simulink model "NCS_Simulation"  (R2019a)
settings: Solver=ode4  StartTime=0.0  StopTime=200  FixedStep=0.004  MaxStep=0.01  RelTol=1e-3
values from neighbouring files (symbols this model uses):
  CAN2EthernetDelay = 0.000    (= 0)    [Parameter.m]
  CycleTime_Sensor = 1/1000    (= 0.001)    [Parameter.m]
  Ethernet2CANDelay = 0.005    [Parameter.m]
  n = 0.001    [Parameter.m]
  nW_ges = 8    [Parameter.m]
  ReferenceDelay = 0.0    (= 0)    [Parameter.m]
undefined symbols (not defined in the file or in its folder): BUSCapacity, controlGate, entity, m, ReadData, ReadSize, v0
libraries: NCS_Library x250, simulink x12
(part 2 of 3)

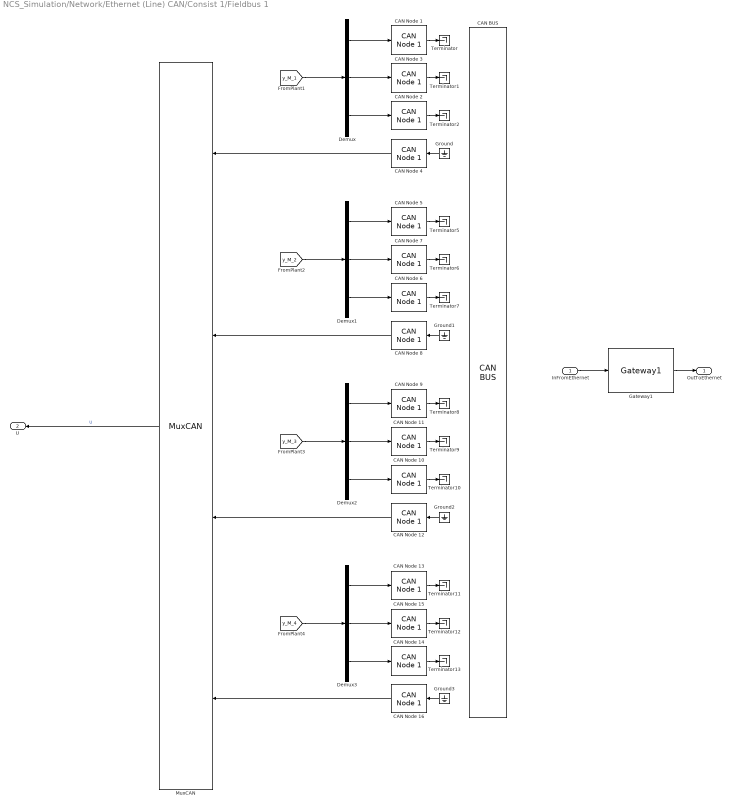
== system NCS_Simulation/Network/Ethernet (Line) CAN/Consist 1/Fieldbus 1 ==
  InFromEthernet : Inport
  CAN BUS : NCS_Library/Network/CAN/CAN BUS  BusID=1  Capacity=500000  LossRate=0.001
  CAN Node 1 : NCS_Library/Network/CAN/CAN Node 1  MsgID=1  IDRange=[1:25]  T_Tx=0.05  SensorType=Position Sensor  MsgSize=8  IDSubscription=[0,0,0,0,0,0,0,0,0,0,0,0,0,0,0,0,0,0,0,0,0,0,0,0,0]  EnableToF=off  ToF=0
  CAN Node 10 : NCS_Library/Network/CAN/CAN Node 1  MsgID=11  IDRange=[1:25]  T_Tx=0.05  SensorType=Acceleration Sensor  MsgSize=8  IDSubscription=[0,0,0,0,0,0,0,0,0,0,0,0,0,0,0,0,0,0,0,0,0,0,0,0,0]  EnableToF=off  ToF=0
  CAN Node 11 : NCS_Library/Network/CAN/CAN Node 1  MsgID=10  IDRange=[1:25]  T_Tx=0.05  SensorType=Velocity Sensor  MsgSize=8  IDSubscription=[0,0,0,0,0,0,0,0,0,0,0,0,0,0,0,0,0,0,0,0,0,0,0,0,0]  EnableToF=off  ToF=0
  CAN Node 12 : NCS_Library/Network/CAN/CAN Node 1  MsgID=12  IDRange=[1:25]  T_Tx=0  SensorType=Actuator  MsgSize=8  IDSubscription=[0,0,0,0,0,0,0,0,0,0,0,0,0,0,0,0,0,0,0,0,0,0,0,0,1]  EnableToF=off  ToF=0
  CAN Node 13 : NCS_Library/Network/CAN/CAN Node 1  MsgID=13  IDRange=[1:25]  T_Tx=0.05  SensorType=Position Sensor  MsgSize=8  IDSubscription=[0,0,0,0,0,0,0,0,0,0,0,0,0,0,0,0,0,0,0,0,0,0,0,0,0]  EnableToF=off  ToF=0
  CAN Node 14 : NCS_Library/Network/CAN/CAN Node 1  MsgID=15  IDRange=[1:25]  T_Tx=0.05  SensorType=Acceleration Sensor  MsgSize=8  IDSubscription=[0,0,0,0,0,0,0,0,0,0,0,0,0,0,0,0,0,0,0,0,0,0,0,0,0]  EnableToF=off  ToF=0
  CAN Node 15 : NCS_Library/Network/CAN/CAN Node 1  MsgID=14  IDRange=[1:25]  T_Tx=0.05  SensorType=Velocity Sensor  MsgSize=8  IDSubscription=[0,0,0,0,0,0,0,0,0,0,0,0,0,0,0,0,0,0,0,0,0,0,0,0,0]  EnableToF=off  ToF=0
  CAN Node 16 : NCS_Library/Network/CAN/CAN Node 1  MsgID=16  IDRange=[1:25]  T_Tx=0  SensorType=Actuator  MsgSize=8  IDSubscription=[0,0,0,0,0,0,0,0,0,0,0,0,0,0,0,0,0,0,0,0,0,0,0,0,1]  EnableToF=off  ToF=0
  CAN Node 2 : NCS_Library/Network/CAN/CAN Node 1  MsgID=3  IDRange=[1:25]  T_Tx=0.05  SensorType=Acceleration Sensor  MsgSize=8  IDSubscription=[0,0,0,0,0,0,0,0,0,0,0,0,0,0,0,0,0,0,0,0,0,0,0,0,0]  EnableToF=off  ToF=0
  CAN Node 3 : NCS_Library/Network/CAN/CAN Node 1  MsgID=2  IDRange=[1:25]  T_Tx=0.05  SensorType=Velocity Sensor  MsgSize=8  IDSubscription=[0,0,0,0,0,0,0,0,0,0,0,0,0,0,0,0,0,0,0,0,0,0,0,0,0]  EnableToF=off  ToF=0
  CAN Node 4 : NCS_Library/Network/CAN/CAN Node 1  MsgID=4  IDRange=[1:25]  T_Tx=0  SensorType=Actuator  MsgSize=8  IDSubscription=[0,0,0,0,0,0,0,0,0,0,0,0,0,0,0,0,0,0,0,0,0,0,0,0,1]  EnableToF=off  ToF=0
  CAN Node 5 : NCS_Library/Network/CAN/CAN Node 1  MsgID=5  IDRange=[1:25]  T_Tx=0.05  SensorType=Position Sensor  MsgSize=8  IDSubscription=[0,0,0,0,0,0,0,0,0,0,0,0,0,0,0,0,0,0,0,0,0,0,0,0,0]  EnableToF=off  ToF=0
  CAN Node 6 : NCS_Library/Network/CAN/CAN Node 1  MsgID=7  IDRange=[1:25]  T_Tx=0.05  SensorType=Acceleration Sensor  MsgSize=8  IDSubscription=[0,0,0,0,0,0,0,0,0,0,0,0,0,0,0,0,0,0,0,0,0,0,0,0,0]  EnableToF=off  ToF=0
  CAN Node 7 : NCS_Library/Network/CAN/CAN Node 1  MsgID=6  IDRange=[1:25]  T_Tx=0.05  SensorType=Velocity Sensor  MsgSize=8  IDSubscription=[0,0,0,0,0,0,0,0,0,0,0,0,0,0,0,0,0,0,0,0,0,0,0,0,0]  EnableToF=off  ToF=0
  CAN Node 8 : NCS_Library/Network/CAN/CAN Node 1  MsgID=8  IDRange=[1:25]  T_Tx=0  SensorType=Actuator  MsgSize=8  IDSubscription=[0,0,0,0,0,0,0,0,0,0,0,0,0,0,0,0,0,0,0,0,0,0,0,0,1]  EnableToF=off  ToF=0
  CAN Node 9 : NCS_Library/Network/CAN/CAN Node 1  MsgID=9  IDRange=[1:25]  T_Tx=0.05  SensorType=Position Sensor  MsgSize=8  IDSubscription=[0,0,0,0,0,0,0,0,0,0,0,0,0,0,0,0,0,0,0,0,0,0,0,0,0]  EnableToF=off  ToF=0
  Demux{,1..3} (4 alike) : Demux  Outputs=3
  Gateway1 : NCS_Library/Network/Gateway/Gateway1  T_Tx=4  MaxNum=8  Address=[111 211]  Destination=[111 200]  Port=1  ReplyAddress=[0 0]  Subscribe=[111 212; 111 213; 0 0; 0 0; 0 0]  Timeout=inf  SDTv2=Disable  SensorType=0  MsgID=25  IDRange=[1:25]  T_Tx_CAN=0.1  MsgSize=8  IDSubscription=[0,1,0,0,0,1,0,0,0,1,0,0,0,1,0,0,0,0,0,0,0,0,0,0,0]  EnableToF=off  ToF=0
  Ground{,1..3} (4 alike) : Ground
  MuxCAN : NCS_Library/Network/Applications/Multiplexer/MuxCAN  SystemSampleTime=-1
  Terminator{,1..2,5..13} (12 alike) : Terminator
  OutToEthernet : Outport
  U : Outport  Port=2
  wires:
  CAN Node 8/1 -> MuxCAN/2
  CAN Node 4/1 -> MuxCAN/1
  Demux/1 -> CAN Node 1/1
  CAN Node 16/1 -> MuxCAN/4
  CAN Node 9/1 -> Terminator8/1
  CAN Node 1/1 -> Terminator/1
  Demux/2 -> CAN Node 3/1
  [y_M_1] -> Demux/1
  Demux3/1 -> CAN Node 13/1
  CAN Node 12/1 -> MuxCAN/3
  Demux2/2 -> CAN Node 11/1
  CAN Node 3/1 -> Terminator1/1
  CAN Node 6/1 -> Terminator7/1
  Ground/1 -> CAN Node 4/1
  CAN Node 5/1 -> Terminator5/1
  Demux/3 -> CAN Node 2/1
  Demux1/3 -> CAN Node 6/1
  Ground3/1 -> CAN Node 16/1
  Ground1/1 -> CAN Node 8/1
  CAN Node 10/1 -> Terminator10/1
  InFromEthernet/1 -> Gateway1/1
  Demux2/1 -> CAN Node 9/1
  CAN Node 11/1 -> Terminator9/1
  CAN Node 13/1 -> Terminator11/1
  Demux2/3 -> CAN Node 10/1
  Demux1/2 -> CAN Node 7/1
  Demux3/2 -> CAN Node 15/1
  CAN Node 14/1 -> Terminator13/1
  Ground2/1 -> CAN Node 12/1
  [y_M_4] -> Demux3/1
  [y_M_3] -> Demux2/1
  Demux1/1 -> CAN Node 5/1
  CAN Node 15/1 -> Terminator12/1
  [y_M_2] -> Demux1/1
  CAN Node 2/1 -> Terminator2/1
  Demux3/3 -> CAN Node 14/1
  CAN Node 7/1 -> Terminator6/1
  MuxCAN/1 -> U/1  "U"
  Gateway1/1 -> OutToEthernet/1

== system NCS_Simulation/Network/Ethernet (Line) CAN/Consist 1/Output Control ==
  <#Receive> : Inport
  Y_M1 : Inport  Port=2
  U : Inport  Port=3
  Y_M2 : Inport  Port=4
  Logical Operator : Logic  Operator=NOT  AllPortsSameDT=off  OutDataTypeStr=boolean
  Mux : NCS_Library/Network/Applications/Multiplexer/Mux  SystemSampleTime=-1
  Switch : Switch  Criteria=u2 > Threshold
  Watch Dog : NCS_Library/Network/Applications/Watch Dog  SystemSampleTime=-1
  Out1 : Outport
  wires:
  Mux/1 -> Out1/1
  Watch Dog/1 -> Logical Operator/1
  U/1 -> Mux/2
  <#Receive>/1 -> Watch Dog/1
  Switch/1 -> Mux/1
  Y_M1/1 -> Switch/1
  Logical Operator/1 -> Switch/2
  Y_M2/1 -> Switch/3

== system NCS_Simulation/Network/Ethernet (Line) CAN/Consist 1/Redundant Device Control ==
  <#Receive> : Inport
  InTx : Inport  Port=2
  Add Constant : Bias  Bias=1
  Display : Display
  Entity Output Switch : EntityOutputSwitch  InputPortMessageModes=m,m  OutputPortMessageModes=m,m  SwitchingCriterion=From control port  SwitchAttributeName=Attribute1
      settings: InputPortMap=u0,u1
  Message Send : MessageSend  OutputPortMessageModes=m
      settings: InputPortMap=u1
  No Failure : EntityTerminator  InputPortMessageModes=m  NumberEntitiesArrived=on
      settings: OutputPortMap=o0
  Watch Dog : NCS_Library/Network/Applications/Watch Dog  SystemSampleTime=-1
  OutTx : Outport
  wires:
  Message Send/1 -> Entity Output Switch/1
  Add Constant/1 -> Message Send/1
  Watch Dog/1 -> Add Constant/1
  No Failure/1 -> Display/1
  <#Receive>/1 -> Watch Dog/1
  Entity Output Switch/1 -> No Failure/1
  InTx/1 -> Entity Output Switch/2
  Entity Output Switch/2 -> OutTx/1

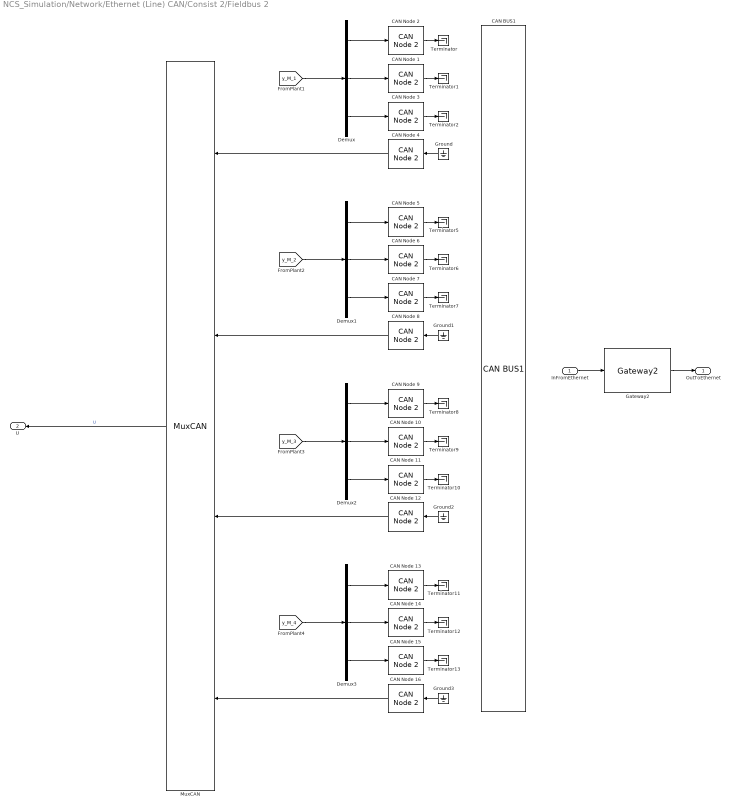
== system NCS_Simulation/Network/Ethernet (Line) CAN/Consist 2/Fieldbus 2 ==
  InFromEthernet : Inport
  CAN BUS1 : NCS_Library/Network/CAN/CAN BUS1  BusID=2  Capacity=500000  LossRate=0.001
  CAN Node 1 : NCS_Library/Network/CAN/CAN Node 2  MsgID=2  IDRange=[1:25]  T_Tx=0.05  SensorType=Velocity Sensor  MsgSize=8  IDSubscription=[0,0,0,0,0,0,0,0,0,0,0,0,0,0,0,0,0,0,0,0,0,0,0,0,0]  EnableToF=off  ToF=0
  CAN Node 10 : NCS_Library/Network/CAN/CAN Node 2  MsgID=10  IDRange=[1:25]  T_Tx=0.05  SensorType=Velocity Sensor  MsgSize=8  IDSubscription=[0,0,0,0,0,0,0,0,0,0,0,0,0,0,0,0,0,0,0,0,0,0,0,0,0]  EnableToF=off  ToF=0
  CAN Node 11 : NCS_Library/Network/CAN/CAN Node 2  MsgID=11  IDRange=[1:25]  T_Tx=0.05  SensorType=Acceleration Sensor  MsgSize=8  IDSubscription=[0,0,0,0,0,0,0,0,0,0,0,0,0,0,0,0,0,0,0,0,0,0,0,0,0]  EnableToF=off  ToF=0
  CAN Node 12 : NCS_Library/Network/CAN/CAN Node 2  MsgID=12  IDRange=[1:25]  T_Tx=0  SensorType=Actuator  MsgSize=8  IDSubscription=[0,0,0,0,0,0,0,0,0,0,0,0,0,0,0,0,0,0,0,0,0,0,0,0,1]  EnableToF=off  ToF=0
  CAN Node 13 : NCS_Library/Network/CAN/CAN Node 2  MsgID=13  IDRange=[1:25]  T_Tx=0.05  SensorType=Position Sensor  MsgSize=8  IDSubscription=[0,0,0,0,0,0,0,0,0,0,0,0,0,0,0,0,0,0,0,0,0,0,0,0,0]  EnableToF=off  ToF=0
  CAN Node 14 : NCS_Library/Network/CAN/CAN Node 2  MsgID=14  IDRange=[1:25]  T_Tx=0.05  SensorType=Velocity Sensor  MsgSize=8  IDSubscription=[0,0,0,0,0,0,0,0,0,0,0,0,0,0,0,0,0,0,0,0,0,0,0,0,0]  EnableToF=off  ToF=0
  CAN Node 15 : NCS_Library/Network/CAN/CAN Node 2  MsgID=15  IDRange=[1:25]  T_Tx=0.05  SensorType=Acceleration Sensor  MsgSize=8  IDSubscription=[0,0,0,0,0,0,0,0,0,0,0,0,0,0,0,0,0,0,0,0,0,0,0,0,0]  EnableToF=off  ToF=0
  CAN Node 16 : NCS_Library/Network/CAN/CAN Node 2  MsgID=16  IDRange=[1:25]  T_Tx=0  SensorType=Actuator  MsgSize=8  IDSubscription=[0,0,0,0,0,0,0,0,0,0,0,0,0,0,0,0,0,0,0,0,0,0,0,0,1]  EnableToF=off  ToF=0
  CAN Node 2 : NCS_Library/Network/CAN/CAN Node 2  MsgID=1  IDRange=[1:25]  T_Tx=0.05  SensorType=Position Sensor  MsgSize=8  IDSubscription=[0,0,0,0,0,0,0,0,0,0,0,0,0,0,0,0,0,0,0,0,0,0,0,0,0]  EnableToF=off  ToF=0
  CAN Node 3 : NCS_Library/Network/CAN/CAN Node 2  MsgID=3  IDRange=[1:25]  T_Tx=0.05  SensorType=Acceleration Sensor  MsgSize=8  IDSubscription=[0,0,0,0,0,0,0,0,0,0,0,0,0,0,0,0,0,0,0,0,0,0,0,0,0]  EnableToF=off  ToF=0
  CAN Node 4 : NCS_Library/Network/CAN/CAN Node 2  MsgID=4  IDRange=[1:25]  T_Tx=0  SensorType=Actuator  MsgSize=8  IDSubscription=[0,0,0,0,0,0,0,0,0,0,0,0,0,0,0,0,0,0,0,0,0,0,0,0,1]  EnableToF=off  ToF=0
  CAN Node 5 : NCS_Library/Network/CAN/CAN Node 2  MsgID=5  IDRange=[1:25]  T_Tx=0.05  SensorType=Position Sensor  MsgSize=8  IDSubscription=[0,0,0,0,0,0,0,0,0,0,0,0,0,0,0,0,0,0,0,0,0,0,0,0,0]  EnableToF=off  ToF=0
  CAN Node 6 : NCS_Library/Network/CAN/CAN Node 2  MsgID=6  IDRange=[1:25]  T_Tx=0.05  SensorType=Velocity Sensor  MsgSize=8  IDSubscription=[0,0,0,0,0,0,0,0,0,0,0,0,0,0,0,0,0,0,0,0,0,0,0,0,0]  EnableToF=off  ToF=0
  CAN Node 7 : NCS_Library/Network/CAN/CAN Node 2  MsgID=7  IDRange=[1:25]  T_Tx=0.05  SensorType=Actuator  MsgSize=8  IDSubscription=[0,0,0,0,0,0,0,0,0,0,0,0,0,0,0,0,0,0,0,0,0,0,0,0,0]  EnableToF=off  ToF=0
  CAN Node 8 : NCS_Library/Network/CAN/CAN Node 2  MsgID=8  IDRange=[1:25]  T_Tx=0  SensorType=Actuator  MsgSize=8  IDSubscription=[0,0,0,0,0,0,0,0,0,0,0,0,0,0,0,0,0,0,0,0,0,0,0,0,1]  EnableToF=off  ToF=0
  CAN Node 9 : NCS_Library/Network/CAN/CAN Node 2  MsgID=9  IDRange=[1:25]  T_Tx=0.05  SensorType=Position Sensor  MsgSize=8  IDSubscription=[0,0,0,0,0,0,0,0,0,0,0,0,0,0,0,0,0,0,0,0,0,0,0,0,0]  EnableToF=off  ToF=0
  Demux{,1..3} (4 alike) : Demux  Outputs=3
  Gateway2 : NCS_Library/Network/Gateway/Gateway2  T_Tx=4  MaxNum=8  Address=[112 211]  Destination=[112 200]  Port=1  ReplyAddress=[0 0]  Subscribe=[112 212; 112 213; 0 0; 0 0; 0 0]  Timeout=inf  SDTv2=Disable  SensorType=0  MsgID=25  IDRange=[1:25]  T_Tx_CAN=0.1  MsgSize=8  IDSubscription=[0,1,0,0,0,1,0,0,0,1,0,0,0,1,0,0,0,0,0,0,0,0,0,0,0]  EnableToF=off  ToF=0
  Ground{,1..3} (4 alike) : Ground
  MuxCAN : NCS_Library/Network/Applications/Multiplexer/MuxCAN  SystemSampleTime=-1
  Terminator{,1..2,5..13} (12 alike) : Terminator
  OutToEthernet : Outport
  U : Outport  Port=2
  wires:
  MuxCAN/1 -> U/1  "U"
  Demux1/2 -> CAN Node 6/1
  Demux/3 -> CAN Node 3/1
  [y_M_2] -> Demux1/1
  Demux3/2 -> CAN Node 14/1
  [y_M_3] -> Demux2/1
  [y_M_4] -> Demux3/1
  Demux3/3 -> CAN Node 15/1
  Demux3/1 -> CAN Node 13/1
  Demux2/2 -> CAN Node 10/1
  InFromEthernet/1 -> Gateway2/1
  Demux2/3 -> CAN Node 11/1
  Demux1/1 -> CAN Node 5/1
  Demux1/3 -> CAN Node 7/1
  Demux/2 -> CAN Node 1/1
  Ground2/1 -> CAN Node 12/1
  [y_M_1] -> Demux/1
  CAN Node 2/1 -> Terminator/1
  Demux2/1 -> CAN Node 9/1
  Ground3/1 -> CAN Node 16/1
  Demux/1 -> CAN Node 2/1
  Ground/1 -> CAN Node 4/1
  Ground1/1 -> CAN Node 8/1
  CAN Node 1/1 -> Terminator1/1
  CAN Node 3/1 -> Terminator2/1
  CAN Node 4/1 -> MuxCAN/1
  CAN Node 5/1 -> Terminator5/1
  CAN Node 6/1 -> Terminator6/1
  CAN Node 7/1 -> Terminator7/1
  CAN Node 8/1 -> MuxCAN/2
  CAN Node 9/1 -> Terminator8/1
  CAN Node 10/1 -> Terminator9/1
  CAN Node 11/1 -> Terminator10/1
  CAN Node 12/1 -> MuxCAN/3
  CAN Node 13/1 -> Terminator11/1
  CAN Node 14/1 -> Terminator12/1
  CAN Node 15/1 -> Terminator13/1
  CAN Node 16/1 -> MuxCAN/4
  Gateway2/1 -> OutToEthernet/1

== system NCS_Simulation/Network/Ethernet (Line) CAN/Consist 2/Output Control ==
  <#Receive> : Inport
  Y_M1 : Inport  Port=2
  U : Inport  Port=3
  Y_M2 : Inport  Port=4
  Logical Operator : Logic  Operator=NOT  AllPortsSameDT=off  OutDataTypeStr=boolean
  MATLAB Function : MATLAB Function  TreatAsAtomicUnit=on
  Switch : Switch  Criteria=u2 > Threshold
  Watch Dog : NCS_Library/Network/Applications/Watch Dog  SystemSampleTime=-1
  Out1 : Outport
  wires:
  Y_M2/1 -> Switch/3
  Logical Operator/1 -> Switch/2
  Y_M1/1 -> Switch/1
  Switch/1 -> MATLAB Function/1(in_Y_M)
  <#Receive>/1 -> Watch Dog/1
  U/1 -> MATLAB Function/2(in_U)
  Watch Dog/1 -> Logical Operator/1
  MATLAB Function/1(out) -> Out1/1

== system NCS_Simulation/Network/Ethernet (Line) CAN/Consist 2/Redundant Device Control ==
  <#Receive> : Inport
  InTx : Inport  Port=2
  Add Constant : Bias  Bias=1
  Display : Display
  Entity Output Switch : EntityOutputSwitch  InputPortMessageModes=m,m  OutputPortMessageModes=m,m  SwitchingCriterion=From control port  SwitchAttributeName=Attribute1
      settings: InputPortMap=u0,u1
  Message Send : MessageSend  OutputPortMessageModes=m
      settings: InputPortMap=u1
  No Failure : EntityTerminator  InputPortMessageModes=m  NumberEntitiesArrived=on
      settings: OutputPortMap=o0
  Watch Dog : NCS_Library/Network/Applications/Watch Dog  SystemSampleTime=-1
  OutTx : Outport
  wires:
  Entity Output Switch/2 -> OutTx/1
  InTx/1 -> Entity Output Switch/2
  Entity Output Switch/1 -> No Failure/1
  <#Receive>/1 -> Watch Dog/1
  No Failure/1 -> Display/1
  Watch Dog/1 -> Add Constant/1
  Add Constant/1 -> Message Send/1
  Message Send/1 -> Entity Output Switch/1

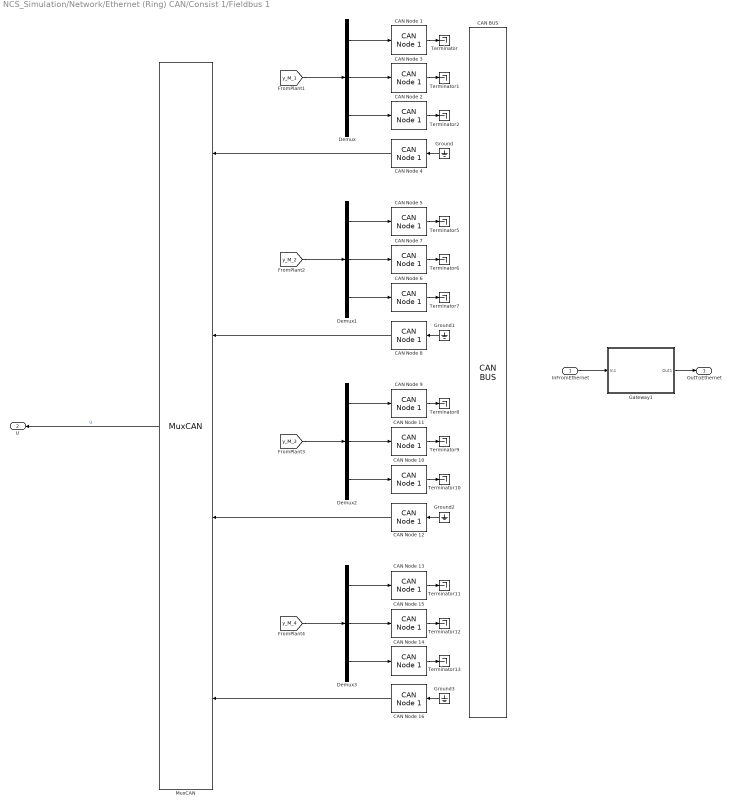
== system NCS_Simulation/Network/Ethernet (Ring) CAN/Consist 1/Fieldbus 1 ==
  InFromEthernet : Inport
  CAN BUS : NCS_Library/Network/CAN/CAN BUS  BusID=1  Capacity=500000  LossRate=0.001
  CAN Node 1 : NCS_Library/Network/CAN/CAN Node 1  MsgID=1  IDRange=[1:25]  T_Tx=0.05  SensorType=Position Sensor  MsgSize=8  IDSubscription=[0,0,0,0,0,0,0,0,0,0,0,0,0,0,0,0,0,0,0,0,0,0,0,0,0]  EnableToF=off  ToF=0
  CAN Node 10 : NCS_Library/Network/CAN/CAN Node 1  MsgID=11  IDRange=[1:25]  T_Tx=0.05  SensorType=Acceleration Sensor  MsgSize=8  IDSubscription=[0,0,0,0,0,0,0,0,0,0,0,0,0,0,0,0,0,0,0,0,0,0,0,0,0]  EnableToF=off  ToF=0
  CAN Node 11 : NCS_Library/Network/CAN/CAN Node 1  MsgID=10  IDRange=[1:25]  T_Tx=0.05  SensorType=Velocity Sensor  MsgSize=8  IDSubscription=[0,0,0,0,0,0,0,0,0,0,0,0,0,0,0,0,0,0,0,0,0,0,0,0,0]  EnableToF=off  ToF=0
  CAN Node 12 : NCS_Library/Network/CAN/CAN Node 1  MsgID=12  IDRange=[1:25]  T_Tx=0  SensorType=Actuator  MsgSize=8  IDSubscription=[0,0,0,0,0,0,0,0,0,0,0,0,0,0,0,0,0,0,0,0,0,0,0,0,1]  EnableToF=off  ToF=0
  CAN Node 13 : NCS_Library/Network/CAN/CAN Node 1  MsgID=13  IDRange=[1:25]  T_Tx=0.05  SensorType=Position Sensor  MsgSize=8  IDSubscription=[0,0,0,0,0,0,0,0,0,0,0,0,0,0,0,0,0,0,0,0,0,0,0,0,0]  EnableToF=off  ToF=0
  CAN Node 14 : NCS_Library/Network/CAN/CAN Node 1  MsgID=15  IDRange=[1:25]  T_Tx=0.05  SensorType=Acceleration Sensor  MsgSize=8  IDSubscription=[0,0,0,0,0,0,0,0,0,0,0,0,0,0,0,0,0,0,0,0,0,0,0,0,0]  EnableToF=off  ToF=0
  CAN Node 15 : NCS_Library/Network/CAN/CAN Node 1  MsgID=14  IDRange=[1:25]  T_Tx=0.05  SensorType=Velocity Sensor  MsgSize=8  IDSubscription=[0,0,0,0,0,0,0,0,0,0,0,0,0,0,0,0,0,0,0,0,0,0,0,0,0]  EnableToF=off  ToF=0
  CAN Node 16 : NCS_Library/Network/CAN/CAN Node 1  MsgID=16  IDRange=[1:25]  T_Tx=0  SensorType=Actuator  MsgSize=8  IDSubscription=[0,0,0,0,0,0,0,0,0,0,0,0,0,0,0,0,0,0,0,0,0,0,0,0,1]  EnableToF=off  ToF=0
  CAN Node 2 : NCS_Library/Network/CAN/CAN Node 1  MsgID=3  IDRange=[1:25]  T_Tx=0.05  SensorType=Acceleration Sensor  MsgSize=8  IDSubscription=[0,0,0,0,0,0,0,0,0,0,0,0,0,0,0,0,0,0,0,0,0,0,0,0,0]  EnableToF=off  ToF=0
  CAN Node 3 : NCS_Library/Network/CAN/CAN Node 1  MsgID=2  IDRange=[1:25]  T_Tx=0.05  SensorType=Velocity Sensor  MsgSize=8  IDSubscription=[0,0,0,0,0,0,0,0,0,0,0,0,0,0,0,0,0,0,0,0,0,0,0,0,0]  EnableToF=off  ToF=0
  CAN Node 4 : NCS_Library/Network/CAN/CAN Node 1  MsgID=4  IDRange=[1:25]  T_Tx=0  SensorType=Actuator  MsgSize=8  IDSubscription=[0,0,0,0,0,0,0,0,0,0,0,0,0,0,0,0,0,0,0,0,0,0,0,0,1]  EnableToF=off  ToF=0
  CAN Node 5 : NCS_Library/Network/CAN/CAN Node 1  MsgID=5  IDRange=[1:25]  T_Tx=0.05  SensorType=Position Sensor  MsgSize=8  IDSubscription=[0,0,0,0,0,0,0,0,0,0,0,0,0,0,0,0,0,0,0,0,0,0,0,0,0]  EnableToF=off  ToF=0
  CAN Node 6 : NCS_Library/Network/CAN/CAN Node 1  MsgID=7  IDRange=[1:25]  T_Tx=0.05  SensorType=Acceleration Sensor  MsgSize=8  IDSubscription=[0,0,0,0,0,0,0,0,0,0,0,0,0,0,0,0,0,0,0,0,0,0,0,0,0]  EnableToF=off  ToF=0
  CAN Node 7 : NCS_Library/Network/CAN/CAN Node 1  MsgID=6  IDRange=[1:25]  T_Tx=0.05  SensorType=Velocity Sensor  MsgSize=8  IDSubscription=[0,0,0,0,0,0,0,0,0,0,0,0,0,0,0,0,0,0,0,0,0,0,0,0,0]  EnableToF=off  ToF=0
  CAN Node 8 : NCS_Library/Network/CAN/CAN Node 1  MsgID=8  IDRange=[1:25]  T_Tx=0  SensorType=Actuator  MsgSize=8  IDSubscription=[0,0,0,0,0,0,0,0,0,0,0,0,0,0,0,0,0,0,0,0,0,0,0,0,1]  EnableToF=off  ToF=0
  CAN Node 9 : NCS_Library/Network/CAN/CAN Node 1  MsgID=9  IDRange=[1:25]  T_Tx=0.05  SensorType=Position Sensor  MsgSize=8  IDSubscription=[0,0,0,0,0,0,0,0,0,0,0,0,0,0,0,0,0,0,0,0,0,0,0,0,0]  EnableToF=off  ToF=0
  Demux{,1..3} (4 alike) : Demux  Outputs=3
  Gateway1 : Subsystem  AncestorBlock=NCS_Library/Network/Gateway/Gateway1  mask{T_Tx=0.1, MaxNum=8, Address=[133 211], Destination=[100 200], Port=1, ReplyAddress=[0 0], Subscribe=[122 211; 144 211; 0 0; 0 0; 0 0], Timeout=inf, SDTv2=Disable, SensorType=0, MsgID=25, IDRange=[1:25], T_Tx_CAN=0.05, MsgSize=8, IDSubscription=[0,1,0,0,0,1,0,0,0,1,0,0,0,1,0,0,0,0,0,0,0,0,0,0,0], EnableToF=off, ToF=0}
      mask prompts: Port "Destination Port"; ReplyAddress "Reply Address"; MsgID "CAN ID"; IDRange "Range of all IDs"; T_Tx_CAN "T_Tx"; MsgSize "DataSIze (0-8 Bytes)"; IDSubscription "IDs of messages subscribed to accept (0-no, 1-yes)"; EnableToF "Failure"; ToF "Time [s]"
      mask TypeOptions Port: 1 | 2 | 3 | 4 | 5 | 6 | 7 | 8 | Multicast
      mask TypeOptions SDTv2: Disable | Enable
      mask Callback EnableToF:
      | % Control parameter visiblity
      | % Disable Tx dialog, if it is not needed, because of a passive ED,
      | % which only receives.
      | 
      | % Get value
      | ToF = get_param(gcb,'EnableToF');
      | % ToB = get_param(gcb,'EnableBurst');
      | 
      | 
      | % Set the 'MaskVisibilities' property for each box
      | 
      | On = {'on','on','on','on','on','on','on','on','on','on','on','on','on','on','on','on','on'}; % Init
      | 
      | % Disable Tx Dialog, if not needed
      | if strcmp('off',ToF)
      |     On{17} = 'off';
      | end
      | 
      | set_param(gcb,'MaskEnables',On );
      mask DialogControl ParameterGroupVar Prompt: Parameters Gateway
      mask DialogControl Container5 Prompt: Parameters Ethernet Interface
      mask DialogControl Container6 Prompt: SDTv2
      mask DialogControl Container3 Prompt: Paramters CAN Interface
      mask DialogControl Container4 Prompt: Interupts
      mask Display: disp( ['Address: ', get_param(gcb,'Address'), '\n \n Ethernet-CAN-Gateway', '\n \n CAN-ID: ', get_param(gcb,'msgID')] )
  Ground{,1..3} (4 alike) : Ground
  MuxCAN : NCS_Library/Network/Applications/Multiplexer/MuxCAN  SystemSampleTime=-1
  Terminator{,1..2,5..13} (12 alike) : Terminator
  OutToEthernet : Outport
  U : Outport  Port=2
  wires:
  CAN Node 8/1 -> MuxCAN/2
  CAN Node 4/1 -> MuxCAN/1
  Demux/1 -> CAN Node 1/1
  CAN Node 16/1 -> MuxCAN/4
  CAN Node 9/1 -> Terminator8/1
  CAN Node 1/1 -> Terminator/1
  Demux/2 -> CAN Node 3/1
  [y_M_1] -> Demux/1
  Demux3/1 -> CAN Node 13/1
  CAN Node 12/1 -> MuxCAN/3
  Demux2/2 -> CAN Node 11/1
  CAN Node 3/1 -> Terminator1/1
  CAN Node 6/1 -> Terminator7/1
  Ground/1 -> CAN Node 4/1
  CAN Node 5/1 -> Terminator5/1
  Demux/3 -> CAN Node 2/1
  Demux1/3 -> CAN Node 6/1
  Ground3/1 -> CAN Node 16/1
  Ground1/1 -> CAN Node 8/1
  CAN Node 10/1 -> Terminator10/1
  InFromEthernet/1 -> Gateway1/1(In1)
  Demux2/1 -> CAN Node 9/1
  CAN Node 11/1 -> Terminator9/1
  CAN Node 13/1 -> Terminator11/1
  Demux2/3 -> CAN Node 10/1
  Demux1/2 -> CAN Node 7/1
  Demux3/2 -> CAN Node 15/1
  CAN Node 14/1 -> Terminator13/1
  Ground2/1 -> CAN Node 12/1
  [y_M_4] -> Demux3/1
  [y_M_3] -> Demux2/1
  Demux1/1 -> CAN Node 5/1
  CAN Node 15/1 -> Terminator12/1
  [y_M_2] -> Demux1/1
  CAN Node 2/1 -> Terminator2/1
  Demux3/3 -> CAN Node 14/1
  CAN Node 7/1 -> Terminator6/1
  MuxCAN/1 -> U/1  "U"
  Gateway1/1(Out1) -> OutToEthernet/1

== system NCS_Simulation/Network/Ethernet (Ring) CAN/Consist 1/Output Control ==
  Failed : Inport
  Y_M1 : Inport  Port=2
  U : Inport  Port=3
  Y_M2 : Inport  Port=4
  Logical Operator : Logic  Operator=NOT  AllPortsSameDT=off  OutDataTypeStr=boolean
  Mux : NCS_Library/Network/Applications/Multiplexer/Mux  SystemSampleTime=-1
  Switch : Switch  Criteria=u2 > Threshold
  Out1 : Outport
  wires:
  Y_M2/1 -> Switch/3
  Logical Operator/1 -> Switch/2
  Y_M1/1 -> Switch/1
  Switch/1 -> Mux/1
  U/1 -> Mux/2
  Failed/1 -> Logical Operator/1
  Mux/1 -> Out1/1

== system NCS_Simulation/Network/Ethernet (Ring) CAN/Consist 1/Redundant Device Control1 ==
  Failed : Inport
  InTx : Inport  Port=2
  Add Constant : Bias  Bias=1
  Display : Display
  Entity Output Switch : EntityOutputSwitch  InputPortMessageModes=m,m  OutputPortMessageModes=m,m  SwitchingCriterion=From control port  SwitchAttributeName=Attribute1
      settings: InputPortMap=u0,u1
  Message Send : MessageSend  OutputPortMessageModes=m
      settings: InputPortMap=u1
  No Failure : EntityTerminator  InputPortMessageModes=m  NumberEntitiesArrived=on
      settings: OutputPortMap=o0
  OutTx : Outport
  wires:
  Entity Output Switch/2 -> OutTx/1
  InTx/1 -> Entity Output Switch/2
  Entity Output Switch/1 -> No Failure/1
  No Failure/1 -> Display/1
  Failed/1 -> Add Constant/1
  Add Constant/1 -> Message Send/1
  Message Send/1 -> Entity Output Switch/1

== system NCS_Simulation/Network/Ethernet (Ring) CAN/Consist 2/ED ==
  RxFromBus : Inport
  Signal : Inport  Port=2
  Clock : Clock
  Compare To Constant : simulink/Logic and Bit Operations/Compare To Constant  relop=>=  const=ToF  OutDataTypeStr=uint8
  Constant : Constant  Value=EnableToF
  Data Type Conversion : DataTypeConversion  OutDataTypeStr=uint8
  Display1 : Display
  Display2 : Display
  Failure Control Rx : NCS_Library/Network/Applications/Failure Control  SystemSampleTime=-1
  Failure Control Tx : NCS_Library/Network/Applications/Failure Control  SystemSampleTime=-1
  Logical Operator : Logic  AllPortsSameDT=off  OutDataTypeStr=boolean
  Protocol Stack : Subsystem
  User Interface : Subsystem
  TxToBus : Outport
  ReceivedData : Outport  Port=2
  Recorder : Outport  Port=3
  Failed : Outport  Port=4
  wires:
  User Interface/1(Parameter) -> Protocol Stack/2(Parameter)
  Failure Control Tx/1 -> TxToBus/1
  Failure Control Rx/1 -> Protocol Stack/3(RxFromBus)
  Protocol Stack/3(TxToBus) -> Failure Control Tx/1
  RxFromBus/1 -> Failure Control Rx/1
  Signal/1 -> Protocol Stack/1(Signal)
  Protocol Stack/1(Data) -> ReceivedData/1
  Protocol Stack/2(Recorder) -> Recorder/1
  Data Type Conversion/1 -> Failed/1
  Constant/1 -> Logical Operator/2
  Clock/1 -> Compare To Constant/1
  Logical Operator/1 -> Display2/1, Data Type Conversion/1
  Compare To Constant/1 -> Display1/1, Logical Operator/1

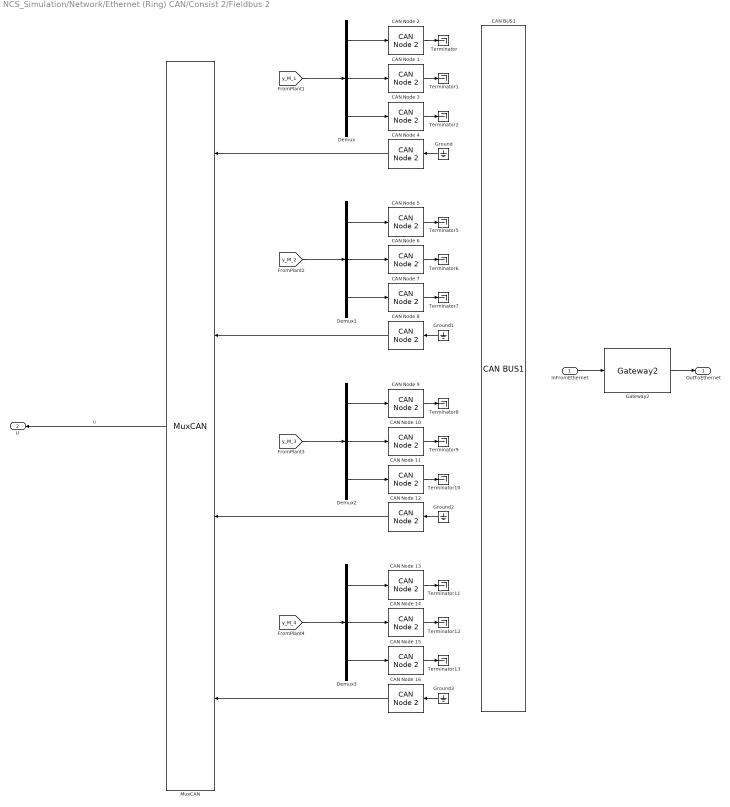
== system NCS_Simulation/Network/Ethernet (Ring) CAN/Consist 2/Fieldbus 2 ==
  InFromEthernet : Inport
  CAN BUS1 : NCS_Library/Network/CAN/CAN BUS1  BusID=2  Capacity=500000  LossRate=0.001
  CAN Node 1 : NCS_Library/Network/CAN/CAN Node 2  MsgID=2  IDRange=[1:25]  T_Tx=0.05  SensorType=Velocity Sensor  MsgSize=8  IDSubscription=[0,0,0,0,0,0,0,0,0,0,0,0,0,0,0,0,0,0,0,0,0,0,0,0,0]  EnableToF=off  ToF=0
  CAN Node 10 : NCS_Library/Network/CAN/CAN Node 2  MsgID=10  IDRange=[1:25]  T_Tx=0.05  SensorType=Velocity Sensor  MsgSize=8  IDSubscription=[0,0,0,0,0,0,0,0,0,0,0,0,0,0,0,0,0,0,0,0,0,0,0,0,0]  EnableToF=off  ToF=0
  CAN Node 11 : NCS_Library/Network/CAN/CAN Node 2  MsgID=11  IDRange=[1:25]  T_Tx=0.05  SensorType=Acceleration Sensor  MsgSize=8  IDSubscription=[0,0,0,0,0,0,0,0,0,0,0,0,0,0,0,0,0,0,0,0,0,0,0,0,0]  EnableToF=off  ToF=0
  CAN Node 12 : NCS_Library/Network/CAN/CAN Node 2  MsgID=12  IDRange=[1:25]  T_Tx=0  SensorType=Actuator  MsgSize=8  IDSubscription=[0,0,0,0,0,0,0,0,0,0,0,0,0,0,0,0,0,0,0,0,0,0,0,0,1]  EnableToF=off  ToF=0
  CAN Node 13 : NCS_Library/Network/CAN/CAN Node 2  MsgID=13  IDRange=[1:25]  T_Tx=0.05  SensorType=Position Sensor  MsgSize=8  IDSubscription=[0,0,0,0,0,0,0,0,0,0,0,0,0,0,0,0,0,0,0,0,0,0,0,0,0]  EnableToF=off  ToF=0
  CAN Node 14 : NCS_Library/Network/CAN/CAN Node 2  MsgID=14  IDRange=[1:25]  T_Tx=0.05  SensorType=Velocity Sensor  MsgSize=8  IDSubscription=[0,0,0,0,0,0,0,0,0,0,0,0,0,0,0,0,0,0,0,0,0,0,0,0,0]  EnableToF=off  ToF=0
  CAN Node 15 : NCS_Library/Network/CAN/CAN Node 2  MsgID=15  IDRange=[1:25]  T_Tx=0.05  SensorType=Acceleration Sensor  MsgSize=8  IDSubscription=[0,0,0,0,0,0,0,0,0,0,0,0,0,0,0,0,0,0,0,0,0,0,0,0,0]  EnableToF=off  ToF=0
  CAN Node 16 : NCS_Library/Network/CAN/CAN Node 2  MsgID=16  IDRange=[1:25]  T_Tx=0  SensorType=Actuator  MsgSize=8  IDSubscription=[0,0,0,0,0,0,0,0,0,0,0,0,0,0,0,0,0,0,0,0,0,0,0,0,1]  EnableToF=off  ToF=0
  CAN Node 2 : NCS_Library/Network/CAN/CAN Node 2  MsgID=1  IDRange=[1:25]  T_Tx=0.05  SensorType=Position Sensor  MsgSize=8  IDSubscription=[0,0,0,0,0,0,0,0,0,0,0,0,0,0,0,0,0,0,0,0,0,0,0,0,0]  EnableToF=off  ToF=0
  CAN Node 3 : NCS_Library/Network/CAN/CAN Node 2  MsgID=3  IDRange=[1:25]  T_Tx=0.05  SensorType=Acceleration Sensor  MsgSize=8  IDSubscription=[0,0,0,0,0,0,0,0,0,0,0,0,0,0,0,0,0,0,0,0,0,0,0,0,0]  EnableToF=off  ToF=0
  CAN Node 4 : NCS_Library/Network/CAN/CAN Node 2  MsgID=4  IDRange=[1:25]  T_Tx=0  SensorType=Actuator  MsgSize=8  IDSubscription=[0,0,0,0,0,0,0,0,0,0,0,0,0,0,0,0,0,0,0,0,0,0,0,0,1]  EnableToF=off  ToF=0
  CAN Node 5 : NCS_Library/Network/CAN/CAN Node 2  MsgID=5  IDRange=[1:25]  T_Tx=0.05  SensorType=Position Sensor  MsgSize=8  IDSubscription=[0,0,0,0,0,0,0,0,0,0,0,0,0,0,0,0,0,0,0,0,0,0,0,0,0]  EnableToF=off  ToF=0
  CAN Node 6 : NCS_Library/Network/CAN/CAN Node 2  MsgID=6  IDRange=[1:25]  T_Tx=0.05  SensorType=Velocity Sensor  MsgSize=8  IDSubscription=[0,0,0,0,0,0,0,0,0,0,0,0,0,0,0,0,0,0,0,0,0,0,0,0,0]  EnableToF=off  ToF=0
  CAN Node 7 : NCS_Library/Network/CAN/CAN Node 2  MsgID=7  IDRange=[1:25]  T_Tx=0.05  SensorType=Actuator  MsgSize=8  IDSubscription=[0,0,0,0,0,0,0,0,0,0,0,0,0,0,0,0,0,0,0,0,0,0,0,0,0]  EnableToF=off  ToF=0
  CAN Node 8 : NCS_Library/Network/CAN/CAN Node 2  MsgID=8  IDRange=[1:25]  T_Tx=0  SensorType=Actuator  MsgSize=8  IDSubscription=[0,0,0,0,0,0,0,0,0,0,0,0,0,0,0,0,0,0,0,0,0,0,0,0,1]  EnableToF=off  ToF=0
  CAN Node 9 : NCS_Library/Network/CAN/CAN Node 2  MsgID=9  IDRange=[1:25]  T_Tx=0.05  SensorType=Position Sensor  MsgSize=8  IDSubscription=[0,0,0,0,0,0,0,0,0,0,0,0,0,0,0,0,0,0,0,0,0,0,0,0,0]  EnableToF=off  ToF=0
  Demux{,1..3} (4 alike) : Demux  Outputs=3
  Gateway2 : NCS_Library/Network/Gateway/Gateway2  T_Tx=4  MaxNum=8  Address=[112 211]  Destination=[112 200]  Port=1  ReplyAddress=[0 0]  Subscribe=[112 212; 112 213; 0 0; 0 0; 0 0]  Timeout=inf  SDTv2=Disable  SensorType=0  MsgID=25  IDRange=[1:25]  T_Tx_CAN=0.1  MsgSize=8  IDSubscription=[0,1,0,0,0,1,0,0,0,1,0,0,0,1,0,0,0,0,0,0,0,0,0,0,0]  EnableToF=off  ToF=0
  Ground{,1..3} (4 alike) : Ground
  MuxCAN : NCS_Library/Network/Applications/Multiplexer/MuxCAN  SystemSampleTime=-1
  Terminator{,1..2,5..13} (12 alike) : Terminator
  OutToEthernet : Outport
  U : Outport  Port=2
  wires:
  MuxCAN/1 -> U/1  "U"
  Demux1/2 -> CAN Node 6/1
  Demux/3 -> CAN Node 3/1
  [y_M_2] -> Demux1/1
  Demux3/2 -> CAN Node 14/1
  [y_M_3] -> Demux2/1
  [y_M_4] -> Demux3/1
  Demux3/3 -> CAN Node 15/1
  Demux3/1 -> CAN Node 13/1
  Demux2/2 -> CAN Node 10/1
  InFromEthernet/1 -> Gateway2/1
  Demux2/3 -> CAN Node 11/1
  Demux1/1 -> CAN Node 5/1
  Demux1/3 -> CAN Node 7/1
  Demux/2 -> CAN Node 1/1
  Ground2/1 -> CAN Node 12/1
  [y_M_1] -> Demux/1
  CAN Node 2/1 -> Terminator/1
  Demux2/1 -> CAN Node 9/1
  Ground3/1 -> CAN Node 16/1
  Demux/1 -> CAN Node 2/1
  Ground/1 -> CAN Node 4/1
  Ground1/1 -> CAN Node 8/1
  CAN Node 1/1 -> Terminator1/1
  CAN Node 3/1 -> Terminator2/1
  CAN Node 4/1 -> MuxCAN/1
  CAN Node 5/1 -> Terminator5/1
  CAN Node 6/1 -> Terminator6/1
  CAN Node 7/1 -> Terminator7/1
  CAN Node 8/1 -> MuxCAN/2
  CAN Node 9/1 -> Terminator8/1
  CAN Node 10/1 -> Terminator9/1
  CAN Node 11/1 -> Terminator10/1
  CAN Node 12/1 -> MuxCAN/3
  CAN Node 13/1 -> Terminator11/1
  CAN Node 14/1 -> Terminator12/1
  CAN Node 15/1 -> Terminator13/1
  CAN Node 16/1 -> MuxCAN/4
  Gateway2/1 -> OutToEthernet/1

== system NCS_Simulation/Network/Ethernet (Ring) CAN/Consist 2/Output Control ==
  <#Receive> : Inport
  Y_M1 : Inport  Port=2
  U : Inport  Port=3
  Y_M2 : Inport  Port=4
  Logical Operator : Logic  Operator=NOT  AllPortsSameDT=off  OutDataTypeStr=boolean
  MATLAB Function : MATLAB Function  TreatAsAtomicUnit=on
  Switch : Switch  Criteria=u2 > Threshold
  Watch Dog : NCS_Library/Network/Applications/Watch Dog  SystemSampleTime=-1
  Out1 : Outport
  wires:
  Y_M2/1 -> Switch/3
  Logical Operator/1 -> Switch/2
  Y_M1/1 -> Switch/1
  Switch/1 -> MATLAB Function/1(in_Y_M)
  <#Receive>/1 -> Watch Dog/1
  U/1 -> MATLAB Function/2(in_U)
  Watch Dog/1 -> Logical Operator/1
  MATLAB Function/1(out) -> Out1/1

== system NCS_Simulation/Network/Ethernet (Ring) CAN/Consist 2/Redundant Device Control ==
  <#Receive> : Inport
  InTx : Inport  Port=2
  Add Constant : Bias  Bias=1
  Display : Display
  Entity Output Switch : EntityOutputSwitch  InputPortMessageModes=m,m  OutputPortMessageModes=m,m  SwitchingCriterion=From control port  SwitchAttributeName=Attribute1
      settings: InputPortMap=u0,u1
  Message Send : MessageSend  OutputPortMessageModes=m
      settings: InputPortMap=u1
  No Failure : EntityTerminator  InputPortMessageModes=m  NumberEntitiesArrived=on
      settings: OutputPortMap=o0
  Watch Dog : NCS_Library/Network/Applications/Watch Dog  SystemSampleTime=-1
  OutTx : Outport
  wires:
  Entity Output Switch/2 -> OutTx/1
  InTx/1 -> Entity Output Switch/2
  Entity Output Switch/1 -> No Failure/1
  <#Receive>/1 -> Watch Dog/1
  No Failure/1 -> Display/1
  Watch Dog/1 -> Add Constant/1
  Add Constant/1 -> Message Send/1
  Message Send/1 -> Entity Output Switch/1

== system NCS_Simulation/Network/Ethernet (Ring) CAN/Consist 1/Fieldbus 1/Gateway1 ==
  In1 : Inport
  CAN Interface : Subsystem
  Ethernet Interface : Subsystem
  Out1 : Outport
  wires:
  Ethernet Interface/1(TxToBus) -> Out1/1
  In1/1 -> Ethernet Interface/1(RxFromBus)
  Ethernet Interface/2(ReceivedData) -> CAN Interface/1(ReceivedData)
  CAN Interface/1(OutEthernetData) -> Ethernet Interface/2(CANData)

== system NCS_Simulation/Network/Ethernet (Ring) CAN/Consist 2/ED/Protocol Stack ==
  Signal : Inport
  Parameter : Inport  Port=2
  RxFromBus : Inport  Port=3
  Bus Selector : BusSelector  OutputSignals=SDTv2,T_Tx,msgType
  CycleRx : EntityServer  InputPortMessageModes=m  OutputPortMessageModes=m  Capacity=inf  ServiceTimeValue=CycleRx
  CycleTx : EntityServer  InputPortMessageModes=m  OutputPortMessageModes=m  Capacity=inf  ServiceTimeValue=CycleTx  EntryAction=ReadSize(entity.Size);
  Display : Display
  IP : NCS_Library/Network/ETB/OSI Layers/IP  SystemSampleTime=-1
  MAC Controller : NCS_Library/Network/ETB/OSI Layers/MAC Controller  SystemSampleTime=-1
  Multiply : Product
  SDTv2 : NCS_Library/Network/ETB/OSI Layers/SDTv2  SystemSampleTime=-1
  Signal1 : InportShadow
  Simulink Function : Subsystem  TreatAsAtomicUnit=on
  Subsystem : Subsystem
  TRDP PD : NCS_Library/Network/ETB/OSI Layers/TRDP PD  SystemSampleTime=-1
  TRDP Timeout : NCS_Library/Network/Applications/TRDP Timeout  SystemSampleTime=-1
  UDP Single-Port : NCS_Library/Network/ETB/OSI Layers/UDP Single-Port  SystemSampleTime=-1
  Data : Outport
  Recorder : Outport  Port=2
  TxToBus : Outport  Port=3
  wires:
  Simulink Function/1(Out1) -> Display/1
  TRDP Timeout/1 -> [Valid]
  [SDTv2] -> Subsystem/13(SDTv2)  "SDTv2"
  Subsystem/1(Out1) -> Recorder/1
  MAC Controller/3 -> Subsystem/12(Retry)  "Retry"
  MAC Controller/2 -> Subsystem/11(#collision)  "#collision"
  IP/3 -> Subsystem/10(delay)  "delay"
  IP/2 -> Subsystem/9(In9)
  TRDP PD/6 -> Subsystem/8(In8)
  TRDP PD/5 -> Subsystem/7(In7), TRDP Timeout/1
  TRDP PD/4 -> Subsystem/6(In6)
  TRDP PD/3 -> Subsystem/5(In5)
  SDTv2/3 -> Subsystem/4(Phase)  "Phase"
  SDTv2/2 -> Subsystem/3(In3)
  [Valid] -> Multiply/1
  SDTv2/1 -> Multiply/2  "Data"
  Multiply/1 -> Data/1, Subsystem/2(Data)  "Data"
  Signal1/1 -> TRDP PD/2  "Signal"
  CycleTx/1 -> MAC Controller/1
  IP/4 -> CycleTx/1
  MAC Controller/1 -> CycleRx/1
  CycleRx/1 -> IP/3
  RxFromBus/1 -> MAC Controller/3
  UDP Single-Port/2 -> IP/1
  IP/1 -> UDP Single-Port/2
  UDP Single-Port/1 -> TRDP PD/4
  Signal/1 -> Subsystem/1(Signal), SDTv2/1  "Signal"
  Parameter/1 -> Bus Selector/1, IP/2, MAC Controller/2, TRDP PD/3
  TRDP PD/7 -> UDP Single-Port/1
  SDTv2/4 -> TRDP PD/1
  TRDP PD/2 -> SDTv2/6
  Bus Selector/2 -> SDTv2/3  "<T_Tx>"
  TRDP PD/1 -> SDTv2/5
  Bus Selector/3 -> SDTv2/4  "<msgType>"
  MAC Controller/4 -> TxToBus/1
  Bus Selector/1 -> SDTv2/2, [SDTv2]  "<SDTv2>"

== system NCS_Simulation/Network/Ethernet (Ring) CAN/Consist 2/ED/User Interface ==
  note: User defined Parameters
  Add : Sum  Inputs=+-
  Bus Creator : BusCreator  Inputs=8
  Constant : Constant  Value=Address  OutDataTypeStr=uint16
  Constant1 : Constant  Value=Destination  OutDataTypeStr=uint16
  Constant2 : Constant  Value=Tx  OutDataTypeStr=double
  Constant3 : Constant  Value=msgType  OutDataTypeStr=uint8
  Constant4 : Constant  Value=SDTv2  OutDataTypeStr=double
  Constant5 : Constant
  Constant6 : Constant  Value=Port  OutDataTypeStr=uint16
  Constant7 : Constant  Value=ReplyAddress  OutDataTypeStr=uint16
  MATLAB Function : MATLAB Function  TreatAsAtomicUnit=on
  MATLAB Function1 : MATLAB Function  TreatAsAtomicUnit=on
  Subscribe : Constant  Value=Subscribe  OutDataTypeStr=uint16
  Subsystem1 : NCS_Library/Network/ETB/ED/User Interface/Subsystem2  SystemSampleTime=-1
  Subsystem2 : Subsystem
  Subsystem3 : NCS_Library/Network/ETB/ED/User Interface/Subsystem2  SystemSampleTime=-1
  Parameter : Outport
  wires:
  Subsystem3/1 -> Bus Creator/4  "ReplyAddress"
  Subsystem1/1 -> Bus Creator/1  "Address"
  Bus Creator/1 -> Parameter/1
  MATLAB Function1/1(y) -> Bus Creator/3  "Subscribe"
  Add/1 -> Bus Creator/8  "SDTv2"
  Constant4/1 -> Add/1
  Constant5/1 -> Add/2
  Subscribe/1 -> MATLAB Function1/1(u)
  Constant1/1 -> Subsystem2/1(In1)
  Constant6/1 -> Bus Creator/5  "Port"
  Constant7/1 -> Subsystem3/1
  Subsystem2/1(Out1) -> Bus Creator/2  "Destination"
  Constant/1 -> Subsystem1/1
  MATLAB Function/1(msgType) -> Bus Creator/7  "msgType"
  Constant3/1 -> MATLAB Function/1(u)
  Constant2/1 -> Bus Creator/6  "T_Tx"

== system NCS_Simulation/Network/Ethernet (Ring) CAN/Consist 1/Fieldbus 1/Gateway1/CAN Interface ==
  ReceivedData : Inport
  Buffer Overflow : EntityTerminator  InputPortMessageModes=m  NumberEntitiesArrived=on
      settings: OutputPortMap=o0
  CAN Interface : Subsystem
  Display{2..4,9} (4 alike) : Display
  Entity Output Switch : EntityOutputSwitch  InputPortMessageModes=m  OutputPortMessageModes=m,m  SwitchAttributeName=Attribute1
  Entity Gate2 : EntityGate  InputPortMessageModes=m,m  OutputPortMessageModes=m
  Entity Gate3 : EntityGate  InputPortMessageModes=m,m  OutputPortMessageModes=m  OperatingMode=Release gate
  Entity Terminator1 : EntityTerminator  InputPortMessageModes=m  NumberEntitiesArrived=on
      settings: OutputPortMap=o0
  Entry Control : Subsystem
  Gate Control : Subsystem
  Message Send1 : MessageSend  OutputPortMessageModes=m
      settings: InputPortMap=u1
  Multicast Receive Queue : EntityQueue  InputPortMessageModes=m  OutputPortMessageModes=n,m  Capacity=100  EntryAction=ReadData(entity.SensorType,entity.Data);  NumberEntitiesInBlock=on
      settings: OutputPortMap=o1,o5
  Multicast Receive Queue1 : EntityQueue  InputPortMessageModes=m  OutputPortMessageModes=n,m  Capacity=inf  NumberEntitiesInBlock=on
      settings: OutputPortMap=o1,o5
  Read Data : Subsystem  TreatAsAtomicUnit=on
  Save Data : Subsystem
  Transport Delay : TransportDelay  DelayTime=CAN2EthernetDelay
  OutEthernetData : Outport
  wires:
  Transport Delay/1 -> OutEthernetData/1
  ReceivedData/1 -> CAN Interface/1(d_in)
  Save Data/1(OutData) -> Transport Delay/1
  Entity Gate2/1 -> Entity Terminator1/1
  Entity Gate3/1 -> Multicast Receive Queue/1
  Multicast Receive Queue1/2 -> Entity Gate3/2
  Message Send1/1 -> Entity Gate2/1
  Entry Control/1(Out1) -> Entity Gate3/1
  Multicast Receive Queue1/1 -> Display9/1
  Multicast Receive Queue/2 -> Entity Gate2/2
  Multicast Receive Queue/1 -> Gate Control/1(n_packets), Entry Control/2(n_packets), Display4/1
  Entity Output Switch/2 -> Buffer Overflow/1
  Buffer Overflow/1 -> Display2/1
  Entity Output Switch/1 -> Multicast Receive Queue1/1
  Entity Terminator1/1 -> Display3/1
  Read Data/2(Data) -> Save Data/2(Data)
  CAN Interface/1(CAN_Message) -> Entity Output Switch/1
  Read Data/1(Type) -> Save Data/1(Type)
  Gate Control/1(FLUSH) -> Message Send1/1, Entry Control/1(FLUSH), Save Data/3(FLUSH)

== system NCS_Simulation/Network/Ethernet (Ring) CAN/Consist 1/Fieldbus 1/Gateway1/Ethernet Interface ==
  RxFromBus : Inport
  CANData : Inport  Port=2
  Buffer : MATLAB Function  Commented=on  TreatAsAtomicUnit=on
  Display : Display  Commented=on
  Display1 : Display
  Display2 : Display  Commented=on
  Enabled Subsystem : Subsystem  Commented=on  TreatAsAtomicUnit=on
  Failure Control : NCS_Library/Network/Applications/Failure Control  SystemSampleTime=-1
  Failure Control1 : NCS_Library/Network/Applications/Failure Control  SystemSampleTime=-1
  MATLAB Function : MATLAB Function  TreatAsAtomicUnit=on
  Memory : Memory  Commented=on  InitialCondition=zeros(3,100)  InheritSampleTime=on
  Protocol Stack : Subsystem
  Subsystem4 : Subsystem  Commented=on
  Terminator : Terminator
  Transport Delay : TransportDelay  DelayTime=Ethernet2CANDelay
  User Interface : Subsystem
  TxToBus : Outport
  ReceivedData : Outport  Port=2
  wires:
  User Interface/1(Out1) -> Protocol Stack/2(Parameter)
  Subsystem4/1(Push) -> Buffer/2(Push), Display2/1, Enabled Subsystem/Enable
  Protocol Stack/1(Data) -> Transport Delay/1
  Memory/1 -> Buffer/1(updatedBuffer)
  Buffer/1(Buffer) -> Memory/1
  Protocol Stack/2(Recorder) -> Terminator/1
  Protocol Stack/3(TxToBus) -> Failure Control1/1
  RxFromBus/1 -> Failure Control/1
  Failure Control1/1 -> TxToBus/1
  Failure Control/1 -> Protocol Stack/3(RxFromBus)
  CANData/1 -> Protocol Stack/1(Signal)
  Transport Delay/1 -> Display/1, MATLAB Function/1(u)
  MATLAB Function/1(y) -> ReceivedData/1

== system NCS_Simulation/Network/Ethernet (Ring) CAN/Consist 2/ED/Protocol Stack/Simulink Function ==
  f : TriggerPort  TriggerType=function-call  IsSimulinkFunction=on  FunctionName=ReadSize  FunctionVisibility=scoped  VariantControl=(inherit)
  u : ArgIn  DisableCoverage=on  ArgumentName=Size
  Out1 : Outport
  wires:
  u/1 -> Out1/1

== system NCS_Simulation/Network/Ethernet (Ring) CAN/Consist 2/ED/Protocol Stack/Subsystem ==
  Signal : Inport
  Data : Inport  Port=2
  In3 : Inport  Port=3
  Phase : Inport  Port=4
  In5 : Inport  Port=5
  In6 : Inport  Port=6
  In7 : Inport  Port=7
  In8 : Inport  Port=8
  In9 : Inport  Port=9
  delay : Inport  Port=10
  #collision : Inport  Port=11
  Retry : Inport  Port=12
  SDTv2 : Inport  Port=13
  Bus Creator1 : BusCreator  Commented=on  Inputs=13
  Data Type Conversion{,1..6} (7 alike) : DataTypeConversion  OutDataTypeStr=double
  Detect Change : simulink/Logic and Bit Operations/Detect Change  vinit=0  OutDataTypeStr=boolean
  Out1 : Outport
  wires:
  Phase/1 -> Bus Creator1/4
  Retry/1 -> Detect Change/1
  delay/1 -> Bus Creator1/10, Out1/1
  In5/1 -> Data Type Conversion1/1
  In8/1 -> Data Type Conversion2/1
  #collision/1 -> Bus Creator1/11
  In3/1 -> Data Type Conversion3/1
  In9/1 -> Data Type Conversion5/1
  Data/1 -> Bus Creator1/2
  In6/1 -> Data Type Conversion/1
  Detect Change/1 -> Data Type Conversion4/1
  Data Type Conversion4/1 -> Bus Creator1/12  "Retry"
  Data Type Conversion2/1 -> Bus Creator1/8  "msgType_receive"
  Data Type Conversion3/1 -> Bus Creator1/3  "SSC"
  In7/1 -> Data Type Conversion6/1
  Data Type Conversion1/1 -> Bus Creator1/5  "#Transmit"
  Data Type Conversion6/1 -> Bus Creator1/7  "#Receive"
  Data Type Conversion5/1 -> Bus Creator1/9  "#damaged"
  Signal/1 -> Bus Creator1/1
  Data Type Conversion/1 -> Bus Creator1/6  "msgType_transmit"
  SDTv2/1 -> Bus Creator1/13  "SDTv2"

== system NCS_Simulation/Network/Ethernet (Ring) CAN/Consist 2/ED/User Interface/Subsystem2 ==
  In1 : Inport
  MATLAB Function : MATLAB Function  TreatAsAtomicUnit=on
  Out1 : Outport
  wires:
  In1/1 -> MATLAB Function/1(u)
  MATLAB Function/1(y) -> Out1/1

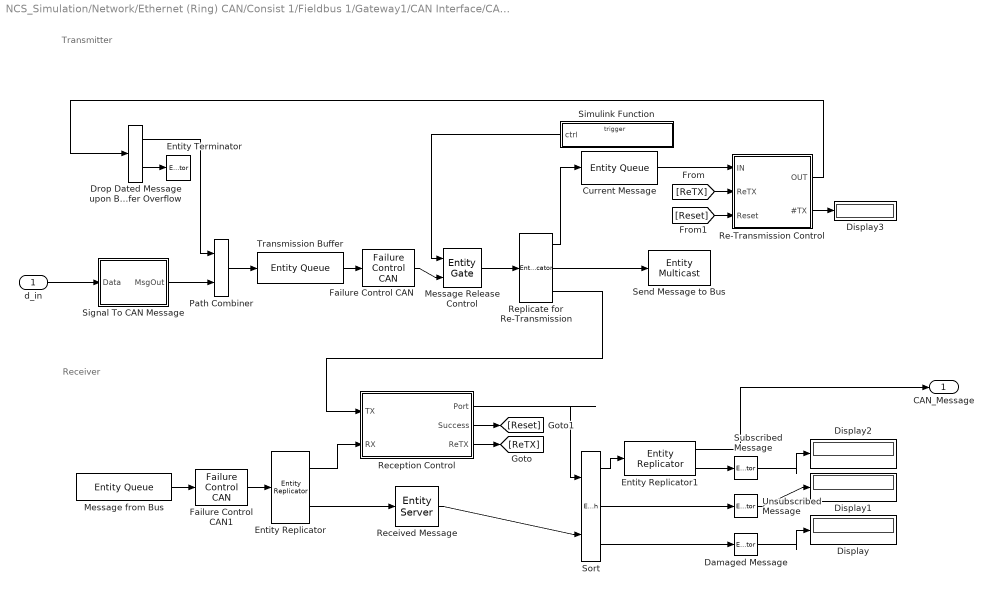
== system NCS_Simulation/Network/Ethernet (Ring) CAN/Consist 1/Fieldbus 1/Gateway1/CAN Interface/CAN Interface ==
  note: Transmitter
  note: Receiver
  d_in : Inport
  Current Message : EntityQueue  InputPortMessageModes=m  OutputPortMessageModes=m  Capacity=2  EntryAction=controlGate(0);  ExitAction=controlGate(1);
      settings: OutputPortMap=o5
  Damaged Message : EntityTerminator  InputPortMessageModes=m  NumberEntitiesArrived=on
      settings: OutputPortMap=o0
  Display{,1..3} (4 alike) : Display
  Drop Dated Message upon Buffer Overflow : EntityOutputSwitch  InputPortMessageModes=m  OutputPortMessageModes=m,m  SwitchAttributeName=Attribute1
  Entity Replicator : EntityReplicator  InputPortMessageModes=m  OutputPortMessageModes=m,m
  Entity Replicator1 : EntityReplicator  InputPortMessageModes=m  OutputPortMessageModes=m,m
  Entity Terminator : EntityTerminator  InputPortMessageModes=m
  Failure Control CAN : NCS_Library/Network/Applications/Failure Control CAN  SystemSampleTime=-1
  Failure Control CAN1 : NCS_Library/Network/Applications/Failure Control CAN  SystemSampleTime=-1
  Message Release Control : EntityGate  InputPortMessageModes=m,m  OutputPortMessageModes=m  OpenGateAtSimulationStart=on
  Message from Bus : EntityQueue  OutputPortMessageModes=m  Capacity=20  EntityArrivalSource=Multicast  MulticastTag=FromBus_1
      settings: OutputPortMap=o5
  Path Combiner : EntityInputSwitch  InputPortMessageModes=m,m  OutputPortMessageModes=m
  Re-Transmission Control : Subsystem
  Received Message : EntityServer  InputPortMessageModes=m  OutputPortMessageModes=m  Capacity=1  ServiceTimeValue=0
  Reception Control : Stateflow chart  TreatAsAtomicUnit=on
  Replicate for Re-Transmission : EntityReplicator  InputPortMessageModes=m  OutputPortMessageModes=m,m,m  NumberReplicas=2
      settings: OutputPortMap=o0,o1,o2
  Send Message to Bus : EntityMulticast  InputPortMessageModes=m  MulticastTag=ToBus_1
  Signal To CAN Message : Subsystem
  Simulink Function : Subsystem  TreatAsAtomicUnit=on
  Sort : EntityOutputSwitch  InputPortMessageModes=m,m  OutputPortMessageModes=m,m,m  NumberOutputPorts=3  SwitchingCriterion=From control port  SwitchAttributeName=Attribute1
      settings: InputPortMap=u0,u1  OutputPortMap=o0,o1,o2
  Subscribed Message : EntityTerminator  InputPortMessageModes=m  NumberEntitiesArrived=on
      settings: OutputPortMap=o0
  Transmission Buffer : EntityQueue  InputPortMessageModes=m  OutputPortMessageModes=m  Capacity=15  QueueType=Priority  PrioritySource=ID
      settings: OutputPortMap=o5
  Unsubscribed Message : EntityTerminator  InputPortMessageModes=m  NumberEntitiesArrived=on
      settings: OutputPortMap=o0
  CAN_Message : Outport
  wires:
  Entity Replicator1/1 -> CAN_Message/1
  Entity Replicator1/2 -> Subscribed Message/1
  Received Message/1 -> Sort/2
  Sort/3 -> Damaged Message/1
  Reception Control/1(Port) -> Sort/1
  Message Release Control/1 -> Replicate for Re-Transmission/1
  Sort/2 -> Unsubscribed Message/1
  [ReTX] -> Re-Transmission Control/2(ReTX)
  Subscribed Message/1 -> Display2/1
  Drop Dated Message upon Buffer Overflow/1 -> Path Combiner/1
  Reception Control/2(Success) -> [Reset]
  Entity Replicator/2 -> Received Message/1
  Signal To CAN Message/1(MsgOut) -> Path Combiner/2
  d_in/1 -> Signal To CAN Message/1(Data)
  Re-Transmission Control/2(#TX) -> Display3/1
  [Reset] -> Re-Transmission Control/3(Reset)
  Damaged Message/1 -> Display/1
  Replicate for Re-Transmission/1 -> Current Message/1
  Path Combiner/1 -> Transmission Buffer/1
  Drop Dated Message upon Buffer Overflow/2 -> Entity Terminator/1
  Unsubscribed Message/1 -> Display1/1
  Failure Control CAN1/1 -> Entity Replicator/1
  Replicate for Re-Transmission/2 -> Send Message to Bus/1
  Entity Replicator/1 -> Reception Control/2(RX)
  Message from Bus/1 -> Failure Control CAN1/1
  Re-Transmission Control/1(OUT) -> Drop Dated Message upon Buffer Overflow/1
  Transmission Buffer/1 -> Failure Control CAN/1
  Reception Control/3(ReTX) -> [ReTX]
  Current Message/1 -> Re-Transmission Control/1(IN)
  Simulink Function/1(ctrl) -> Message Release Control/1
  Replicate for Re-Transmission/3 -> Reception Control/1(TX)
  Failure Control CAN/1 -> Message Release Control/2
  Sort/1 -> Entity Replicator1/1

== system NCS_Simulation/Network/Ethernet (Ring) CAN/Consist 1/Fieldbus 1/Gateway1/CAN Interface/Entry Control ==
  note: refresh
  note: new entity in buffer AND buffer is NOT flushed
  FLUSH : Inport
  n_packets : Inport  Port=2
  Add : Sum
  Add1 : Sum  Inputs=+-
  Compare To Zero : simulink/Logic and Bit Operations/Compare To Zero  relop===  OutDataTypeStr=boolean
  Compare To Zero1 : simulink/Logic and Bit Operations/Compare To Zero  relop=>  OutDataTypeStr=boolean
  Delay : Delay  DelayLength=1  InitialCondition=1
  Display1 : Display
  Enabled Subsystem : Subsystem  TreatAsAtomicUnit=on
  Entity Server : EntityServer  InputPortMessageModes=m  OutputPortMessageModes=n,m  Capacity=1  ServiceTimeValue=0  NumberEntitiesDeparted=on
      settings: OutputPortMap=o0,o9
  FLUSH1 : InportShadow
  Memory : Memory
  Multiply : Product
  Out1 : Outport
  wires:
  Enabled Subsystem/1(Out1) -> Entity Server/1
  Entity Server/2 -> Out1/1
  Entity Server/1 -> Display1/1
  FLUSH1/1 -> Delay/1
  Delay/1 -> Add/2
  Add/1 -> Enabled Subsystem/Enable
  FLUSH/1 -> Compare To Zero/1
  Multiply/1 -> Add/1
  Compare To Zero1/1 -> Multiply/2
  Compare To Zero/1 -> Multiply/1
  Add1/1 -> Compare To Zero1/1
  Memory/1 -> Add1/2
  n_packets/1 -> Memory/1, Add1/1

== system NCS_Simulation/Network/Ethernet (Ring) CAN/Consist 1/Fieldbus 1/Gateway1/CAN Interface/Gate Control ==
  note: Number condition
  note: Time condition
  n_packets : Inport
  Add : Sum  Inputs=-+
  Add2 : Sum
  Add3 : Sum  Inputs=-+-+
  Clock : Clock
  Compare To Zero : simulink/Logic and Bit Operations/Compare To Zero  relop=>=  OutDataTypeStr=uint8
  Compare To Zero1 : simulink/Logic and Bit Operations/Compare To Zero  relop=>=  OutDataTypeStr=uint8
  Compare To Zero2 : simulink/Logic and Bit Operations/Compare To Zero  relop=>  OutDataTypeStr=uint8
  Constant : Constant  Value=T_Tx
  Constant1 : Constant  Value=MaxNum
  Constant2 : Constant  Value=1e-10
  Memory : Memory  InheritSampleTime=on
  Multiply : Product
  Multiply1 : Product
  Save last release time1 : Subsystem
  FLUSH : Outport
  wires:
  Add3/1 -> Compare To Zero1/1
  Save last release time1/1(Out1) -> Memory/1
  Constant2/1 -> Add3/4  "Compensate numeric drift"
  Clock/1 -> Add3/2
  Memory/1 -> Save last release time1/1(Time), Multiply1/1
  Constant/1 -> Add3/3, Multiply1/2  "T_Tx"
  Multiply1/1 -> Add3/1
  Add/1 -> Compare To Zero/1
  Compare To Zero1/1 -> Add2/1
  Constant1/1 -> Add/1
  n_packets/1 -> Compare To Zero2/1, Add/2
  Compare To Zero/1 -> Add2/2
  Add2/1 -> Multiply/1
  Multiply/1 -> FLUSH/1, Save last release time1/Enable
  Compare To Zero2/1 -> Multiply/2

== system NCS_Simulation/Network/Ethernet (Ring) CAN/Consist 1/Fieldbus 1/Gateway1/CAN Interface/Read Data ==
  ReadData : TriggerPort  TriggerType=function-call  IsSimulinkFunction=on  FunctionName=ReadData  FunctionVisibility=scoped  VariantControl=(inherit)
  SensorType : ArgIn  DisableCoverage=on  OutDataTypeStr=uint8  ArgumentName=SensorType
  SensorType1 : ArgIn  DisableCoverage=on  Port=2  ArgumentName=Data
  Type : Outport
  Data : Outport  Port=2  OutputWhenDisabled=reset  InitialOutput=0
  wires:
  SensorType/1 -> Type/1
  SensorType1/1 -> Data/1
